simulink model "SkyGroundSMC"  (R2025b)
settings: Solver=VariableStepAuto  StartTime=0.0  StopTime=10.0  MaxStep=1e-2  RelTol=1e-3
values from neighbouring files (symbols this model uses):
  cb = 0.5    [MPCVariables.mat]    (also in SkyGroundSMCVariables.mat)
  cs = 693.233627451    [MPCVariables.mat]    (also in SkyGroundSMCVariables.mat = 1500)
  Er = 12    [MPCVariables.mat]    (also in SkyGroundSMCVariables.mat)
  gr = -270.361114706    [MPCVariables.mat]    (also in SkyGroundSMCVariables.mat = -186.455941176)
  kb = 0.2    [MPCVariables.mat]    (also in SkyGroundSMCVariables.mat)
  ke = 62.6    [MPCVariables.mat]    (also in SkyGroundSMCVariables.mat)
  ki = 77.9    [MPCVariables.mat]    (also in SkyGroundSMCVariables.mat)
  ks = 5495    [MPCVariables.mat]    (also in SkyGroundSMCVariables.mat)
  kt = 48000    [MPCVariables.mat]    (also in SkyGroundSMCVariables.mat)
  L = 0.0128    [MPCVariables.mat]    (also in SkyGroundSMCVariables.mat)
  L_DC = 0    [MPCVariables.mat]    (also in SkyGroundSMCVariables.mat)
  ms = 82    [MPCVariables.mat]    (also in SkyGroundSMCVariables.mat)
  mu = 11.5    [MPCVariables.mat]    (also in SkyGroundSMCVariables.mat)
  R = 10.2    [MPCVariables.mat]    (also in SkyGroundSMCVariables.mat)
  Rv = 0    [MPCVariables.mat]    (also in SkyGroundSMCVariables.mat)
  sk = 693.233627451    [MPCVariables.mat]    (also in SkyGroundSMCVariables.mat)
settings Model: Creator=khalidwaleed  LastModifiedBy=khalidwaleed
settings SolverCC: ZeroCrossAlgorithm=Adaptive
settings DebuggingCC: MaskedZcDiagnostic=none  IgnoredZcDiagnostic=none

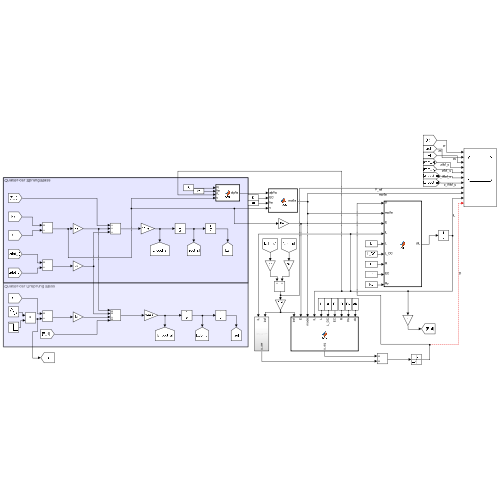
[thumbnail: Simulink's stored preview of the top-level diagram]
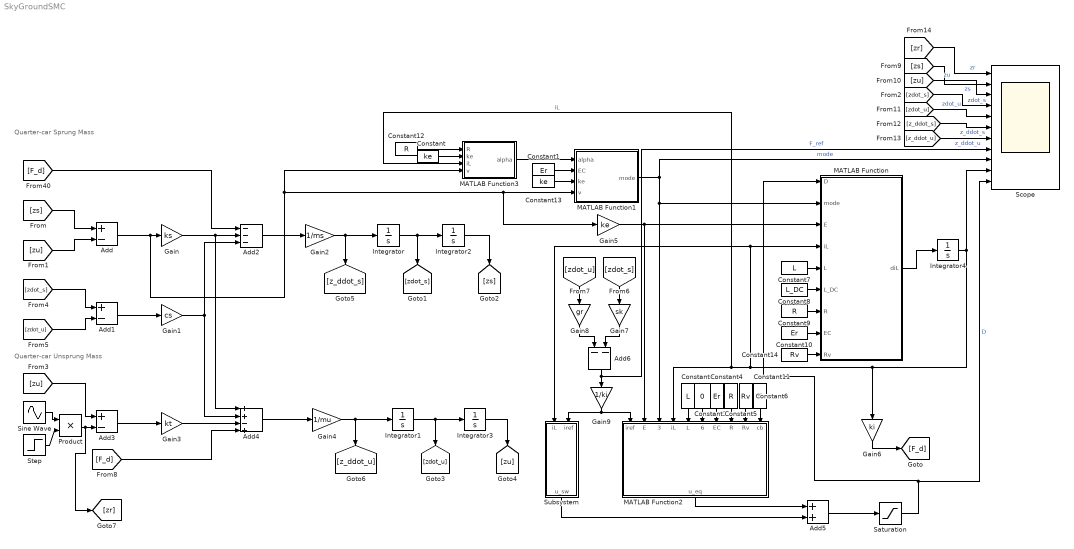
== system SkyGroundSMC ==
  note: Quarter-car Sprung Mass
  note: Quarter-car Unsprung Mass
  Add : Sum  Inputs=+-
  Add1 : Sum  Inputs=+-
  Add2 : Sum  Inputs=---
  Add3 : Sum  Inputs=+-
  Add4 : Sum  Inputs=++-+
  Add5 : Sum
  Add6 : Sum  Inputs=--
  Constant : Constant  Value=ke
  Constant1 : Constant  Value=Er
  Constant10 : Constant  Value=Er
  Constant11 : Constant  Value=cb
  Constant12 : Constant  Value=R
  Constant13 : Constant  Value=ke
  Constant14 : Constant  Value=Rv
  Constant2 : Constant  Value=L
  Constant3 : Constant  Value=0
  Constant4 : Constant  Value=Er
  Constant5 : Constant  Value=R
  Constant6 : Constant  Value=Rv
  Constant7 : Constant  Value=L
  Constant8 : Constant  Value=L_DC
  Constant9 : Constant  Value=R
  Gain : Gain  Gain=ks
  Gain1 : Gain  Gain=cs
  Gain2 : Gain  Gain=1/ms
  Gain3 : Gain  Gain=kt
  Gain4 : Gain  Gain=1/mu
  Gain5 : Gain  Gain=ke
  Gain6 : Gain  Gain=ki
  Gain7 : Gain  Gain=sk
  Gain8 : Gain  Gain=gr
  Gain9 : Gain  Gain=1/ki
  Integrator{,1..4} (5 alike) : Integrator
  MATLAB Function : MATLAB Function  TreatAsAtomicUnit=on
  MATLAB Function1 : MATLAB Function  TreatAsAtomicUnit=on
  MATLAB Function2 : MATLAB Function  TreatAsAtomicUnit=on
  MATLAB Function3 : MATLAB Function  TreatAsAtomicUnit=on
  Product : Product
  Saturation : Saturate  UpperLimit=1  LowerLimit=0
  Scope : Scope  NumInputPorts=11
      settings: ActiveDisplayYMinimum=-0.018748934797028095  ActiveDisplayYMaximum=0.16874041317325289
  Sine Wave : Sin  Amplitude=0.15  Frequency=2*pi  SampleTime=0
  Step : Step  Time=0.48  Before=1  After=0  SampleTime=0
  Subsystem : Subsystem
  wires:
  [zu] -> Add3/1
  Integrator3/1 -> [zu]
  Gain3/1 -> Add4/3
  Add/1 -> MATLAB Function3/4(v), Gain5/1, MATLAB Function1/4(v), Gain/1
  Integrator1/1 -> Integrator3/1, [zdot_u]
  Gain4/1 -> Integrator1/1, [z_ddot_u]
  Gain1/1 -> Add4/2, Add2/3
  Add4/1 -> Gain4/1
  Add2/1 -> Gain2/1
  Gain/1 -> Add4/1, Add2/2
  [zdot_s] -> Add1/1
  [zu] -> Add/2
  Add1/1 -> Gain1/1
  Add3/1 -> Gain3/1
  Integrator2/1 -> [zs]
  Integrator/1 -> Integrator2/1, [zdot_s]
  [zs] -> Add/1
  [zdot_u] -> Add1/2
  Gain2/1 -> Integrator/1, [z_ddot_s]
  Integrator4/1 -> Scope/10, Gain6/1, Subsystem/1(iL), MATLAB Function/4(iL), MATLAB Function3/3(iL), MATLAB Function2/4(iL)  "iL"
  MATLAB Function/1(diL) -> Integrator4/1
  MATLAB Function1/1(mode) -> MATLAB Function2/3(mode), MATLAB Function/2(mode), Scope/9  "mode"
  Gain5/1 -> MATLAB Function2/2(E), MATLAB Function/3(E)
  MATLAB Function2/1(u_eq) -> Add5/1
  Subsystem/1(u_sw) -> Add5/2
  Add5/1 -> Saturation/1
  Saturation/1 -> Scope/11, MATLAB Function/1(D)  "D"
  MATLAB Function3/1(alpha) -> MATLAB Function1/1(alpha)
  Constant/1 -> MATLAB Function3/2(ke)
  Constant1/1 -> MATLAB Function1/2(EC)
  Constant2/1 -> MATLAB Function2/5(L)
  Constant3/1 -> MATLAB Function2/6(L_DC)
  Constant4/1 -> MATLAB Function2/7(EC)
  Constant5/1 -> MATLAB Function2/8(R)
  Constant6/1 -> MATLAB Function2/9(Rv)
  Constant7/1 -> MATLAB Function/5(L)
  Constant8/1 -> MATLAB Function/6(L_DC)
  Constant9/1 -> MATLAB Function/7(R)
  Constant10/1 -> MATLAB Function/8(EC)
  [zdot_s] -> Gain7/1
  [zdot_u] -> Gain8/1
  Gain8/1 -> Add6/1
  Gain7/1 -> Add6/2
  Add6/1 -> Scope/8, Gain9/1  "F_ref"
  Gain9/1 -> MATLAB Function2/1(iref), Subsystem/2(iref)
  Constant11/1 -> MATLAB Function2/10(cb)
  Constant12/1 -> MATLAB Function3/1(R)
  Constant13/1 -> MATLAB Function1/3(ke)
  Constant14/1 -> MATLAB Function/9(Rv)
  [zs] -> Scope/2  "zs"
  [zu] -> Scope/3  "zu"
  [zdot_s] -> Scope/4  "zdot_s"
  [zdot_u] -> Scope/5  "zdot_u"
  [z_ddot_s] -> Scope/6  "z_ddot_s"
  [z_ddot_u] -> Scope/7  "z_ddot_u"
  Gain6/1 -> [F_d]
  Step/1 -> Product/2
  Product/1 -> [zr], Add3/2
  Sine Wave/1 -> Product/1
  [zr] -> Scope/1  "zr"
  [F_d] -> Add2/1
  [F_d] -> Add4/4

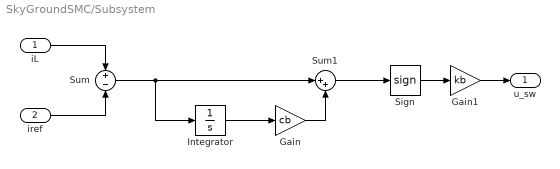
== system SkyGroundSMC/Subsystem ==
  iL : Inport
  iref : Inport  Port=2
  Gain : Gain  Gain=cb
  Gain1 : Gain  Gain=kb
  Integrator : Integrator
  Sign : Signum
  Sum : Sum  Inputs=+-
  Sum1 : Sum  Inputs=|++
  u_sw : Outport
  wires:
  iL/1 -> Sum/1
  iref/1 -> Sum/2
  Sum/1 -> Sum1/1, Integrator/1
  Integrator/1 -> Gain/1
  Gain/1 -> Sum1/2
  Sum1/1 -> Sign/1
  Sign/1 -> Gain1/1
  Gain1/1 -> u_sw/1

== matlab function SkyGroundSMC/MATLAB Function1 ==
  data: alpha input; EC input; ke input; v input; mode output
function mode = mode(alpha, EC, ke, v)
v_alpha = EC/(ke-alpha*ke);
if v<v_alpha
    mode = 1;
else
    mode = 0;
end

== matlab function SkyGroundSMC/MATLAB Function ==
  data: D input; mode input; E input; iL input; diL output; L input; L_DC input; R input; EC input; Rv input
function diL = diL(D, mode, E, iL, L, L_DC, R, EC, Rv)
    LDC = L + L_DC;
    if mode == 1  % boost
        diL = -(R/LDC)*iL - ((1-D)/LDC)*EC + (1/LDC)*E;
    else          % buck
        diL  = -((D*R*L + (1-D)*(R+Rv)*LDC)/(L * LDC))*iL - (D/LDC)*EC + (D*L + (1-D)*LDC)/(L * LDC) * E;
    end
end

== matlab function SkyGroundSMC/MATLAB Function2 ==
  data: iref input; E input; mode input; iL input; u_eq output; L input; L_DC input; EC input; R input; Rv input; cb input
function u_eq = fcn(iref, E, mode, iL, L, L_DC, EC, R, Rv, cb)
    LDC = L + L_DC;
    e   = iL - iref;        % current error

    if mode == 1  % boost
        numerator   = EC - E + R*iref + cb*e*LDC;
        denominator = EC;
        u_eq = numerator / denominator;

    else          % buck
        numerator   = E - (R + Rv)*iref - cb*e*L;
        denominator = (L*R*iref)/LDC - (R + Rv)*iref + ((EC - E)*L)/LDC + E;
        u_eq = numerator / denominator;
    end
end

== matlab function SkyGroundSMC/MATLAB Function3 ==
  data: R input; ke input; iL input; v input; alpha output
function alpha = fcn(R, ke, iL, v)
    i_max = (ke * abs(v)) / R;
    if i_max < 1e-6      % avoid divide-by-zero at v=0
        alpha = 0;
    else
        alpha = abs(iL) / i_max;
    end
end
